simulink model "PlaneFlexSim"  (Simulink 7.4)
settings: Solver=ode23tb  StartTime=0  StopTime=10  FixedStep=ts  MaxStep=.01  RelTol=1e-3
model workspace (MAT data in the model file):
  ts : num (value not decoded)
values from neighbouring files (symbols this model uses):
  simRunner = SimRunner('simRunner')    [testSimRunner.m]
libraries: mblibv1 x23, FlutterLib x8, simulink x1
settings Model: Creator=cstephen  ModifiedByFormat=Rafal  LastModifiedBy=Rafal  ExtModeArmWhenConnect=off  BufferReuse=off
settings DataIOCC: LimitDataPoints=off  SaveOutput=off  SaveTime=off  SignalLoggingName=sigsOut
settings OptimizationCC: BlockReduction=off  InlineParams=on  OptimizeBlockIOStorage=off  BufferReuse=off  EnforceIntegerDowncast=off  ExpressionFolding=off  FoldNonRolledExpr=off  LocalBlockOutputs=off  InitFltsAndDblsToZero=on
settings DebuggingCC: AlgebraicLoopMsg=none  SaveWithParameterizedLinksMsg=none  SignalResolutionControl=TryResolveAllWithWarning  SolverPrmCheckMsg=none  MultiTaskDSMMsg=warning  MultiTaskCondExecSysMsg=none  UnconnectedInputMsg=none  UnconnectedOutputMsg=none  UnconnectedLineMsg=none  StrictBusMsg=None
settings HardwareCC: TargetUnknown=on
settings RTWCC: SystemTargetFile=xpctarget.tlc  TemplateMakefile=xpc_default_tmf  ProcessScript=xpctarget_make_rtw_hook  IncludeERTFirstTime=on
settings xpcTargetCC: TargetFcnLib=ansi_tfl_tmw.mat  TargetFunctionLibrary=ANSI_C  ParMdlRefBuildCompliant=off  CompOptLevelCompliant=off  PortableWordSizes=off
settings CustomProperty: DataType=string  Value=Real-Time
settings SimMechanicsCC: VisDuringSimulation=on  VisSampleTime=0.1  LastVizWinPosition=[360 278 560 420]  CamPosition=[0;-0.208325;16.8123;]  CamTarget=[0;-0.208325;0.424625;]  CamUpVector=[0;1;0;]  CamHeight=4.41673  VisBackgroundColor=[0.9;0.9;0.95;]  DefaultBodyColor=[1;0;0;]

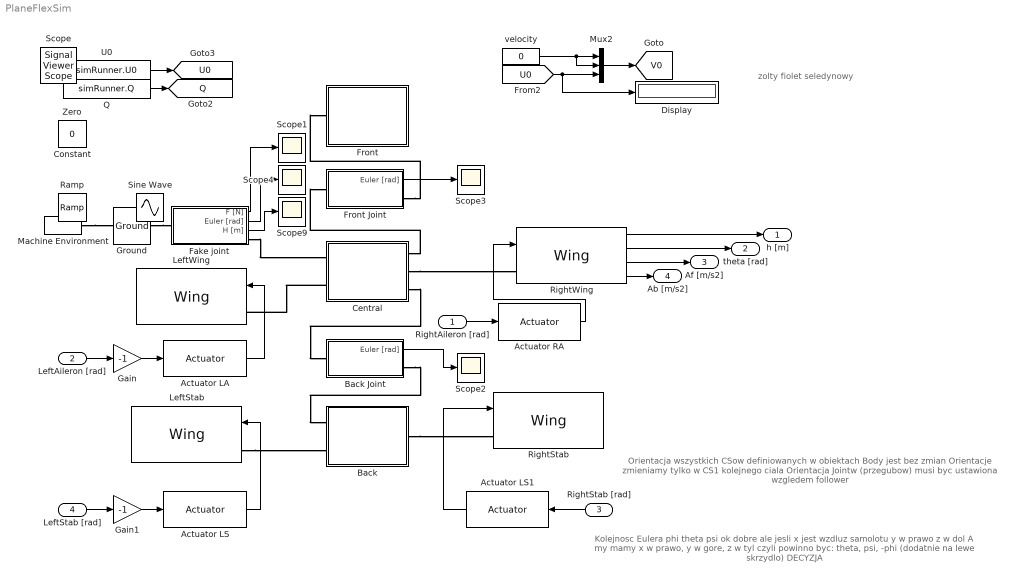
== system PlaneFlexSim ==
  note: Orientacja wszystkich CSow definiowanych
      | w obiektach Body jest bez zmian
      | Orientacje zmieniamy tylko w CS1 kolejnego ciala
      | Orientacja Jointw (przegubow) musi byc ustawiona
      | wzgledem follower
  note: zolty
      | fiolet
      | seledynowy
  note: Kolejnosc Eulera
      | phi theta psi
      | ok dobre ale jesli x jest wzdluz samolotu
      | y w prawo z w dol
      | A my mamy x w prawo, y w gore, z w tyl
      | czyli powinno byc:
      | theta, psi, -phi (dodatnie na lewe skrzydlo)
      | DECYZJA
  RightAileron [rad] : Inport  OutDataType=fixdt(1, 16)  OutScaling=2^0
  LeftAileron [rad] : Inport  Port=2  OutDataType=fixdt(1, 16)  OutScaling=2^0
  RightStab [rad] : Inport  Port=3  OutDataType=fixdt(1, 16)  OutScaling=2^0
  LeftStab [rad] : Inport  Port=4  OutDataType=fixdt(1, 16)  OutScaling=2^0
  Actuator LA : FlutterLib/Actuator  SystemSampleTime=-1  actuator=simRunner.actuator
  Actuator LS : FlutterLib/Actuator  SystemSampleTime=-1  actuator=simRunner.actuator
  Actuator LS1 : FlutterLib/Actuator  SystemSampleTime=-1  actuator=simRunner.actuator
  Actuator RA : FlutterLib/Actuator  SystemSampleTime=-1  actuator=simRunner.actuator
  Back : Subsystem
  Back Joint : Subsystem
  Central : Subsystem
  Display : Display
  Fake joint : Subsystem
  Front : Subsystem
  Front Joint : Subsystem
  Gain : Gain  Gain=-1  ParameterDataType=fixdt(1, 16)  ParameterScaling=2^0  OutDataType=fixdt(1, 16)  OutScaling=2^0
  Gain1 : Gain  Gain=-1  ParameterDataType=fixdt(1, 16)  ParameterScaling=2^0  OutDataType=fixdt(1, 16)  OutScaling=2^0
  Ground : mblibv1/Bodies/Ground  DialogController=MECH.DynMechDlgSource  SystemSampleTime=-1  UpdateFromCAD=off  LeftPortType=env  RightPortType=workingframe  PhysicalDomain=Mechanical  DialogClass=GroundBlock  CoordPosition=[0 0 0]  CoordPositionUnits=m  StateVectorMgrId=-1  MachineId=[0 0]  ShowEnvPort=on
  LeftStab : FlutterLib/Wing  SystemSampleTime=-1  wing=simRunner.stabParams  wingOrientation=[0 0 210]
  LeftWing : FlutterLib/Wing  SystemSampleTime=-1  wing=simRunner.wingParams  wingOrientation=[0 0 -180]
  Machine Environment : mblibv1/Bodies/Machine Environment  DialogController=MECH.DialogSource  SystemSampleTime=-1  PortType=env  PhysicalDomain=Mechanical  DialogTemplateClass=MECH.MachineEnvironment  SyncWhenCopied=off  Gravity=[0 -simRunner.g 0]  GravityUnits=m/s^2  GravityAsSignal=off  Dimensionality=3D Only  AnalysisType=Forward dynamics  LinearAssemblyTolerance=1e-3  LinearAssemblyToleranceUnits=m  AngularAssemblyTolerance=1e-3  AngularAssemblyToleranceUnits=rad  ConstraintSolverType=Stabilizing  ConstraintRelTolerance=1e-4  ConstraintAbsTolerance=1e-4  UseRobustSingularityHandling=off  RedundancyAnalysisToleranceType=Automatically select tolerance  RedundancyAnalysisTolerance=1e-14  StatePerturbationType=Adaptive  PerturbationSize=1e-3  VisualizeMachine=on  BodyVisualizationType=Use model default body geometries  BodyColorSelMode=Use model default  DefaultBodyColor=[1 0 0]
  Mux2 : Mux  Inputs=3
  Q : Constant  Value=simRunner.Q  OutDataType=sfix(16)  OutScaling=2^0
  RightStab : FlutterLib/Wing  SystemSampleTime=-1  wing=simRunner.stabParams  wingOrientation=[0 0 -30]
  RightWing : FlutterLib/Wing  SystemSampleTime=-1  wing=simRunner.wingParams  wingOrientation=[0 0 0]
  Scope{1..4,9} (5 alike) : Scope
      Scope3 settings: SaveName=ScopeData2
      Scope4 settings: SaveName=ScopeData3
      Scope9 settings: SaveName=ScopeData8
  U0 : Constant  Value=simRunner.U0  OutDataType=sfix(16)  OutScaling=2^0
  velocity : Constant  Value=0  OutDataType=sfix(16)  OutScaling=2^0
  h [m] : Outport  OutDataType=fixdt(1, 16)  OutScaling=2^0
  theta [rad] : Outport  Port=2  OutDataType=fixdt(1, 16)  OutScaling=2^0
  Af [m/s2] : Outport  Port=3  OutDataType=fixdt(1, 16)  OutScaling=2^0
  Ab [m/s2] : Outport  Port=4  OutDataType=fixdt(1, 16)  OutScaling=2^0
  Constant : Constant  IOType=siggen  Value=-1  OutDataType=sfix(16)  OutScaling=2^0
  Ramp : simulink/Sources/Ramp  IOType=siggen  SystemSampleTime=-1  slope=1  start=0  X0=0
  Scope : SignalViewerScope  IOType=viewer  ZoomMode=xonly  LegendLocations="674.3333      275.3333            95            41"  RefreshTime=0.035000
      settings: ShowLegends=on  YMin=-0.0018  YMax=0.0002
  Sine Wave : Sin  IOType=siggen  Amplitude=10  Bias=0  Frequency=5  Phase=pi/2  Samples=10  SampleTime=0  Offset=0
  Zero : Constant  IOType=siggen  Value=0  OutDataType=sfix(16)  OutScaling=2^0
  tag scope: Q=global, U0=global, V0=global
  wires:
  [U0] -> Mux2/3, Display/1
  Mux2/1 -> [V0]
  velocity/1 -> Mux2/1, Mux2/2
  Fake joint/1(F [N]) -> Scope1/1
  Front Joint/1(Euler [rad]) -> Scope3/1
  Back Joint/1(Euler [rad]) -> Scope2/1
  Fake joint/2(Euler [rad]) -> Scope4/1
  RightAileron [rad]/1 -> Actuator RA/1
  LeftStab [rad]/1 -> Gain1/1
  RightStab [rad]/1 -> Actuator LS1/1
  Fake joint/3(H [m]) -> Scope9/1
  U0/1 -> [U0]
  Q/1 -> [Q]
  Actuator RA/1 -> RightWing/1
  RightWing/2 -> theta [rad]/1
  RightWing/1 -> h [m]/1
  RightWing/3 -> Af [m/s2]/1
  RightWing/4 -> Ab [m/s2]/1
  LeftAileron [rad]/1 -> Gain/1
  Actuator LA/1 -> LeftWing/1
  Actuator LS/1 -> LeftStab/1
  Actuator LS1/1 -> RightStab/1
  Gain/1 -> Actuator LA/1
  Gain1/1 -> Actuator LS/1
  connections:
  Machine Environment/RConn1 -- Ground/LConn1
  Ground/RConn1 -- Fake joint/LConn1
  Fake joint/RConn1 -- Central/LConn1
  Central/RConn3 -- Back Joint/LConn1
  Back Joint/RConn1 -- Back/LConn1
  Central/RConn1 -- Front Joint/LConn1
  Front Joint/RConn1 -- Front/LConn1
  Back/RConn1 -- RightStab/LConn1
  LeftStab/LConn1 -- Back/LConn2
  Central/LConn2 -- LeftWing/LConn1
  Central/RConn2 -- RightWing/LConn1

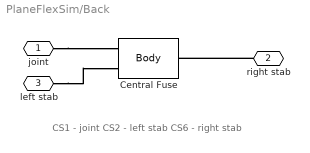
== system PlaneFlexSim/Back ==
  note: CS1 - joint
      | CS2 - left stab
      | CS6 - right stab
  Central Fuse : mblibv1/Bodies/Body  DialogController=MECH.DynMechDlgSource  PhysicalDomain=mechanical  SubClassName=Unknown  LeftPortType=workingframe  RightPortType=workingframe  LConnTagsString=CS1|CS2  RConnTagsString=CS6  UpdateFromCAD=off  DialogClass=MechanicalBodyBlock  Mass=simRunner.fuse.Back.Mass  MassUnits=kg  InertiaUnits=kg*m^2  Inertia=simRunner.fuse.Back.Inertia  Shape=Cylinder  ShapeDims=[1 1]  ShapeUnits=m  ShapeUse=false  Density=1  DensityUnits=kg/m^3  DensityUse=false  GraphicsMode=MACHINE_DEFAULT  BodyColorSelMode=MACHINE_DEFAULT  BodyColor=[1 0 0]  AttachedToCS=CG  CG=Left$CG$simRunner.fuse.Back.CG$CS1$CS1$m$[0 0 0]$Euler X-Y-Z$deg$CS1$false$none  WorkingFrames=Left$CS1$[0 0 0]$Adjoining$Adjoining$m$[0 0 0]$Euler X-Y-Z$deg$Adjoining$true$none#Right$CS6$[0 0 3.1]$CS1$CS1$m$[0 0 0]$Euler X-Y-Z$deg$CS1$true$none#Left$CS2$[0 0 3.1]$CS1$CS1$m$[0 0 0]$Euler X-Y-Z$deg$CS1$true$none#Left$CS5$[-0.4 0 0]$CS1$CS1$m$[0 0 0]$Euler X-Y-Z$deg$CS1$false$none#Left$CS3$[0 0.8 0]$CS1$CS1$m$[0 0 0]$Euler X-Y-Z$deg$CS1$false$none#Left$CS9$[0.4 0 0]$CS1$CS1$m$[0 0 0]$Euler X-Y-Z$deg$CS1$false$none#Left$CS8$[0 -0.2 0]$CS1$CS1$m$[0 0 0]$Euler X-Y-Z$deg$CS1$false$none#Left$CS10$[-0.2 0 3.6]$CS1$CS1$m$[0 0 0]$Euler X-Y-Z$deg$CS1$false$none#Left$CS13$[0 0.2 3.6]$CS1$CS1$m$[0 0 0]$Euler X-Y-Z$deg$CS1$false$none#Left$CS12$[0.2 0 3.6]$CS1$CS1$m$[0 0 0]$Euler X-Y-Z$deg$CS1$false$none#Left$CS11$[0 -0.1 3.6]$CS1$CS1$m$[0 0 0]$Euler X-Y-Z$deg$CS1$false$none  CGPos=simRunner.fuse.Back.CG  CGRot=[0 0 0]  CS0Pos=[]  CS0Rot=[]  CS1Pos=[0 0 0]  CS1Rot=[0 0 0]  CS2Pos=[0 0 3.1]  CS2Rot=[0 0 0]  CS3Pos=[0 0.8 0]  CS3Rot=[0 0 0]  CS4Pos=[]  CS4Rot=[]  CS5Pos=[-0.4 0 0]  CS5Rot=[0 0 0]  CS6Pos=[0 0 3.1]  CS6Rot=[0 0 0]  CS7Pos=[]  CS7Rot=[]  CS8Pos=[0 -0.2 0]  CS8Rot=[0 0 0]  CS9Pos=[0.4 0 0]  CS9Rot=[0 0 0]  CS10Pos=[-0.2 0 3.6]  CS10Rot=[0 0 0]  CS11Pos=[0 -0.1 3.6]  CS11Rot=[0 0 0]  CS12Pos=[0.2 0 3.6]  CS12Rot=[0 0 0]  CS13Pos=[0 0.2 3.6]  CS13Rot=[0 0 0]  CS14Pos=[]  CS14Rot=[]  CS15Pos=[]  CS15Rot=[]  CS16Pos=[]  CS16Rot=[]  CS17Pos=[]  CS17Rot=[]  CS18Pos=[]  CS18Rot=[]  CS19Pos=[]  CS19Rot=[]  CS20Pos=[]  CS20Rot=[]
  joint : PMIOPort  Port=1  Side=Left
  right stab : PMIOPort  Port=2  Side=Right
  left stab : PMIOPort  Port=3  Side=Left
  connections:
  right stab/RConn1 -- Central Fuse/RConn1
  joint/RConn1 -- Central Fuse/LConn1
  left stab/RConn1 -- Central Fuse/LConn2

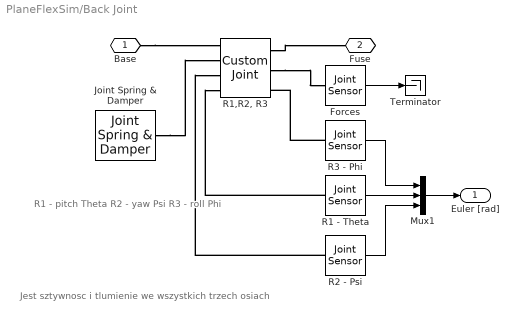
== system PlaneFlexSim/Back Joint ==
  note: R1 - pitch Theta
      | R2 - yaw Psi
      | R3 - roll Phi
  note: Jest sztywnosc i
      | tlumienie
      | we wszystkich trzech
      | osiach
  Forces : mblibv1/Sensors &  Actuators/Joint Sensor  DialogController=MECH.DynMechDlgSource  SystemSampleTime=-1  UpdateFromCAD=off  PhysicalDomain=Mechanical  PortType=blob  Muxed=on  Pose=off  Angle=off  AngleUnits=rad  ArcVelocity=off  ArcVelocityUnits=rad/s  ArcAcceleration=off  ArcAccelerationUnits=deg/s^2  CoordPosition=on  CoordPositionUnits=m  Velocity=off  VelocityUnits=m/s  Acceleration=off  AccelerationUnits=m/s^2  Quaternion=on  QuaternionDT=off  QuaternionDDT=off  QuaternionUnits=off  OutputVector=[1]  ActiveIO=on  Width=3  DialogClass=MechanicalSensorBlock  Primitive=R1  Force=off  ForceUnits=N  Torque=off  TorqueUnits=N*m  ReferenceFrame=Absolute (World)  ReactionSensedSide=Base  ReactionReferenceFrame=Absolute (World)  ReactionForce=on  ReactionForceUnits=N  ReactionMoment=off  ReactionMomentUnits=N*m
  Joint Spring & Damper : mblibv1/Force  Elements/Joint Spring & Damper  DialogController=MECH.DynMechDlgSource  SystemSampleTime=-1  UpdateFromCAD=off  DialogClass=JointSpringDamper  JFEParameters=P1$false$0$0$0$m$m/s$N$deg$deg/s$N*m#P2$false$0$0$0$m$m/s$N$deg$deg/s$N*m#P3$false$0$0$0$m$m/s$N$deg$deg/s$N*m#R1$true$simRunner.fuse.K.K_theta$simRunner.fuse.K.Zeta_theta$0$m$m/s$N$deg$deg/s$N*m#R2$true$simRunner.fuse.K.K_psi$simRunner.fuse.K.Zeta_psi$0$m$m/s$N$deg$deg/s$N*m#R3$true$simRunner.fuse.K.K_phi$simRunner.fuse.K.Zeta_phi$0$m$m/s$N$deg$deg/s$N*m#S$false$0$0$0$m$m/s$N$deg$deg/s$N*m
  Mux1 : Mux  Inputs=3
  R1 - Theta : mblibv1/Sensors &  Actuators/Joint Sensor  DialogController=MECH.DynMechDlgSource  SystemSampleTime=-1  UpdateFromCAD=off  PhysicalDomain=Mechanical  PortType=blob  Muxed=on  Pose=off  Angle=on  AngleUnits=rad  ArcVelocity=off  ArcVelocityUnits=rad/s  ArcAcceleration=off  ArcAccelerationUnits=deg/s^2  CoordPosition=on  CoordPositionUnits=m  Velocity=off  VelocityUnits=m/s  Acceleration=off  AccelerationUnits=m/s^2  Quaternion=on  QuaternionDT=off  QuaternionDDT=off  QuaternionUnits=off  OutputVector=[1]  ActiveIO=on  Width=1  DialogClass=MechanicalSensorBlock  Primitive=R1  Force=off  ForceUnits=N  Torque=off  TorqueUnits=N*m  ReferenceFrame=Absolute (World)  ReactionSensedSide=Base  ReactionReferenceFrame=Absolute (World)  ReactionForce=off  ReactionForceUnits=N  ReactionMoment=off  ReactionMomentUnits=N*m
  "R1,R2, R3" : mblibv1/Joints/Custom Joint  DialogController=MECH.DynMechDlgSource  PhysicalDomain=mechanical  SubClassName=custom_joint  LeftPortType=blob  RightPortType=blob  LConnTagsString=__newl0|SA1|SA2|SA3  RConnTagsString=__newr0|SA1|SA2  UpdateFromCAD=off  NumSAPorts=5  CutJoint=off  MarkAsCut=off  Primitives=prismatic  PrimitiveProps=R1$Follower$[1 0 0]$revolute#R2$Follower$[0 1 0]$Revolute#R3$Follower$[0 0 1]$Revolute  DialogClass=JointBlock  R1Axis=[1 0 0]  R2Axis=[0 1 0]  R3Axis=[0 0 1]  P1Axis=[]  P2Axis=[]  P3Axis=[]  SAxis=[]
  R2 - Psi : mblibv1/Sensors &  Actuators/Joint Sensor  DialogController=MECH.DynMechDlgSource  SystemSampleTime=-1  UpdateFromCAD=off  PhysicalDomain=Mechanical  PortType=blob  Muxed=on  Pose=off  Angle=on  AngleUnits=rad  ArcVelocity=off  ArcVelocityUnits=rad/s  ArcAcceleration=off  ArcAccelerationUnits=deg/s^2  CoordPosition=on  CoordPositionUnits=m  Velocity=off  VelocityUnits=m/s  Acceleration=off  AccelerationUnits=m/s^2  Quaternion=on  QuaternionDT=off  QuaternionDDT=off  QuaternionUnits=off  OutputVector=[1]  ActiveIO=on  Width=1  DialogClass=MechanicalSensorBlock  Primitive=R2  Force=off  ForceUnits=N  Torque=off  TorqueUnits=N*m  ReferenceFrame=Absolute (World)  ReactionSensedSide=Base  ReactionReferenceFrame=Absolute (World)  ReactionForce=off  ReactionForceUnits=N  ReactionMoment=off  ReactionMomentUnits=N*m
  R3 - Phi : mblibv1/Sensors &  Actuators/Joint Sensor  DialogController=MECH.DynMechDlgSource  SystemSampleTime=-1  UpdateFromCAD=off  PhysicalDomain=Mechanical  PortType=blob  Muxed=on  Pose=off  Angle=on  AngleUnits=rad  ArcVelocity=off  ArcVelocityUnits=rad/s  ArcAcceleration=off  ArcAccelerationUnits=deg/s^2  CoordPosition=on  CoordPositionUnits=m  Velocity=off  VelocityUnits=m/s  Acceleration=off  AccelerationUnits=m/s^2  Quaternion=on  QuaternionDT=off  QuaternionDDT=off  QuaternionUnits=off  OutputVector=[1]  ActiveIO=on  Width=1  DialogClass=MechanicalSensorBlock  Primitive=R3  Force=off  ForceUnits=N  Torque=off  TorqueUnits=N*m  ReferenceFrame=Absolute (World)  ReactionSensedSide=Base  ReactionReferenceFrame=Absolute (World)  ReactionForce=off  ReactionForceUnits=N  ReactionMoment=off  ReactionMomentUnits=N*m
  Terminator : Terminator
  Base : PMIOPort  Port=1  Side=Left
  Fuse : PMIOPort  Port=2  Side=Right
  Euler [rad] : Outport  OutDataType=fixdt(1, 16)  OutScaling=2^0
  wires:
  Mux1/1 -> Euler [rad]/1
  R2 - Psi/1 -> Mux1/3
  R1 - Theta/1 -> Mux1/2
  R3 - Phi/1 -> Mux1/1
  Forces/1 -> Terminator/1
  connections:
  R1 - Theta/LConn1 -- "R1,R2, R3"/LConn4
  R3 - Phi/LConn1 -- "R1,R2, R3"/RConn3
  Base/RConn1 -- "R1,R2, R3"/LConn1
  "R1,R2, R3"/RConn1 -- Fuse/RConn1
  "R1,R2, R3"/RConn2 -- Forces/LConn1
  R2 - Psi/LConn1 -- "R1,R2, R3"/LConn3
  Joint Spring & Damper/LConn1 -- "R1,R2, R3"/LConn2

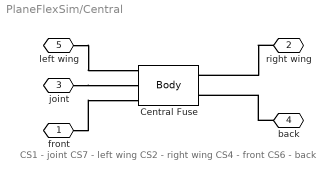
== system PlaneFlexSim/Central ==
  note: CS1 - joint
      | CS7 - left wing
      | CS2 - right wing
      | CS4 - front
      | CS6 - back
  Central Fuse : mblibv1/Bodies/Body  DialogController=MECH.DynMechDlgSource  PhysicalDomain=mechanical  SubClassName=Unknown  LeftPortType=workingframe  RightPortType=workingframe  LConnTagsString=CS7|CS1|CS4  RConnTagsString=CS2|CS6  UpdateFromCAD=off  DialogClass=MechanicalBodyBlock  Mass=simRunner.fuse.Central.Mass  MassUnits=kg  InertiaUnits=kg*m^2  Inertia=simRunner.fuse.Central.Inertia  Shape=Cylinder  ShapeDims=[1 1]  ShapeUnits=m  ShapeUse=false  Density=1  DensityUnits=kg/m^3  DensityUse=false  GraphicsMode=MACHINE_DEFAULT  BodyColorSelMode=MACHINE_DEFAULT  BodyColor=[1 0 0]  AttachedToCS=CG  CG=Left$CG$[0 0 0.3]$CS1$CS1$m$[0 0 0]$Euler X-Y-Z$deg$CS1$false$none  WorkingFrames=Left$CS7$[-0.4 0 0]$CS1$CS1$m$[0 0 0]$Euler X-Y-Z$deg$CS1$true$none#Left$CS1$[0 0 0]$Adjoining$Adjoining$m$[5 0 0]$Euler X-Y-Z$deg$Adjoining$true$none#Right$CS2$[0.4 0 0]$CS1$CS1$m$[0 0 0]$Euler X-Y-Z$deg$CS1$true$none#Left$CS4$[0 0 -0.3]$CS1$CS1$m$[0 0 0]$Euler X-Y-Z$deg$CS1$true$none#Right$CS6$[0 0 0.9]$CS1$CS1$m$[0 0 0]$Euler X-Y-Z$deg$CS1$true$none#Left$CS5$[-0.4 0 -0.3]$CS1$CS1$m$[0 0 0]$Euler X-Y-Z$deg$CS1$false$none#Left$CS3$[0 0.8 -0.3]$CS1$CS1$m$[0 0 0]$Euler X-Y-Z$deg$CS1$false$none#Left$CS9$[0.4 0 -0.3]$CS1$CS1$m$[0 0 0]$Euler X-Y-Z$deg$CS1$false$none#Left$CS8$[0 -0.2 -0.3]$CS1$CS1$m$[0 0 0]$Euler X-Y-Z$deg$CS1$false$none#Left$CS10$[-0.4 0 0.9]$CS1$CS1$m$[0 0 0]$Euler X-Y-Z$deg$CS1$false$none#Left$CS13$[0 0.8 0.9]$CS1$CS1$m$[0 0 0]$Euler X-Y-Z$deg$CS1$false$none#Left$CS12$[0.4 0 0.9]$CS1$CS1$m$[0 0 0]$Euler X-Y-Z$deg$CS1$false$none#Left$CS11$[0 -0.2 0.9]$CS1$CS1$m$[0 0 0]$Euler X-Y-Z$deg$CS1$false$none  CGPos=[0 0 0.3]  CGRot=[0 0 0]  CS0Pos=[]  CS0Rot=[]  CS1Pos=[0 0 0]  CS1Rot=[5 0 0]  CS2Pos=[0.4 0 0]  CS2Rot=[0 0 0]  CS3Pos=[0 0.8 -0.3]  CS3Rot=[0 0 0]  CS4Pos=[0 0 -0.3]  CS4Rot=[0 0 0]  CS5Pos=[-0.4 0 -0.3]  CS5Rot=[0 0 0]  CS6Pos=[0 0 0.9]  CS6Rot=[0 0 0]  CS7Pos=[-0.4 0 0]  CS7Rot=[0 0 0]  CS8Pos=[0 -0.2 -0.3]  CS8Rot=[0 0 0]  CS9Pos=[0.4 0 -0.3]  CS9Rot=[0 0 0]  CS10Pos=[-0.4 0 0.9]  CS10Rot=[0 0 0]  CS11Pos=[0 -0.2 0.9]  CS11Rot=[0 0 0]  CS12Pos=[0.4 0 0.9]  CS12Rot=[0 0 0]  CS13Pos=[0 0.8 0.9]  CS13Rot=[0 0 0]  CS14Pos=[]  CS14Rot=[]  CS15Pos=[]  CS15Rot=[]  CS16Pos=[]  CS16Rot=[]  CS17Pos=[]  CS17Rot=[]  CS18Pos=[]  CS18Rot=[]  CS19Pos=[]  CS19Rot=[]  CS20Pos=[]  CS20Rot=[]
  front : PMIOPort  Port=1  Side=Right
  right wing : PMIOPort  Port=2  Side=Right
  joint : PMIOPort  Port=3  Side=Left
  back : PMIOPort  Port=4  Side=Right
  left wing : PMIOPort  Port=5  Side=Left
  connections:
  left wing/RConn1 -- Central Fuse/LConn1
  right wing/RConn1 -- Central Fuse/RConn1
  joint/RConn1 -- Central Fuse/LConn2
  back/RConn1 -- Central Fuse/RConn2
  front/RConn1 -- Central Fuse/LConn3

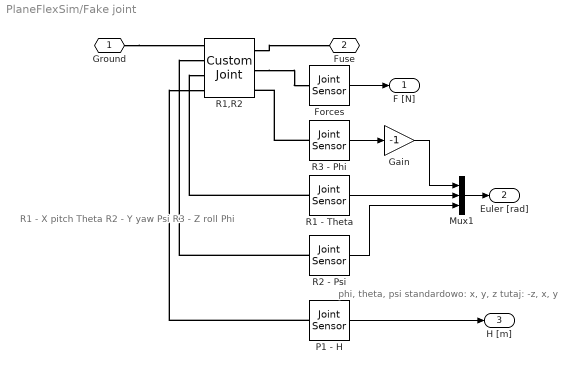
== system PlaneFlexSim/Fake joint ==
  note: R1 - X pitch Theta
      | R2 - Y yaw Psi
      | R3 - Z roll Phi
  note: phi, theta, psi
      | standardowo: x, y, z
      | tutaj: -z, x, y
  Forces : mblibv1/Sensors &  Actuators/Joint Sensor  DialogController=MECH.DynMechDlgSource  SystemSampleTime=-1  UpdateFromCAD=off  PhysicalDomain=Mechanical  PortType=blob  Muxed=on  Pose=off  Angle=off  AngleUnits=rad  ArcVelocity=off  ArcVelocityUnits=rad/s  ArcAcceleration=off  ArcAccelerationUnits=deg/s^2  CoordPosition=on  CoordPositionUnits=m  Velocity=off  VelocityUnits=m/s  Acceleration=off  AccelerationUnits=m/s^2  Quaternion=on  QuaternionDT=off  QuaternionDDT=off  QuaternionUnits=off  OutputVector=[1]  ActiveIO=on  Width=3  DialogClass=MechanicalSensorBlock  Primitive=R1  Force=off  ForceUnits=N  Torque=off  TorqueUnits=N*m  ReferenceFrame=Absolute (World)  ReactionSensedSide=Base  ReactionReferenceFrame=Absolute (World)  ReactionForce=on  ReactionForceUnits=N  ReactionMoment=off  ReactionMomentUnits=N*m
  Gain : Gain  Gain=-1  ParameterDataType=fixdt(1, 16)  ParameterScaling=2^0  OutDataType=fixdt(1, 16)  OutScaling=2^0
  Mux1 : Mux  Inputs=3
  P1 - H : mblibv1/Sensors &  Actuators/Joint Sensor  DialogController=MECH.DynMechDlgSource  SystemSampleTime=-1  UpdateFromCAD=off  PhysicalDomain=Mechanical  PortType=blob  Muxed=on  Pose=off  Angle=off  AngleUnits=rad  ArcVelocity=off  ArcVelocityUnits=rad/s  ArcAcceleration=off  ArcAccelerationUnits=deg/s^2  CoordPosition=on  CoordPositionUnits=m  Velocity=off  VelocityUnits=m/s  Acceleration=off  AccelerationUnits=m/s^2  Quaternion=on  QuaternionDT=off  QuaternionDDT=off  QuaternionUnits=off  OutputVector=[1]  ActiveIO=on  Width=1  DialogClass=MechanicalSensorBlock  Primitive=P1  Force=off  ForceUnits=N  Torque=off  TorqueUnits=N*m  ReferenceFrame=Absolute (World)  ReactionSensedSide=Base  ReactionReferenceFrame=Absolute (World)  ReactionForce=off  ReactionForceUnits=N  ReactionMoment=off  ReactionMomentUnits=N*m
  R1 - Theta : mblibv1/Sensors &  Actuators/Joint Sensor  DialogController=MECH.DynMechDlgSource  SystemSampleTime=-1  UpdateFromCAD=off  PhysicalDomain=Mechanical  PortType=blob  Muxed=on  Pose=off  Angle=on  AngleUnits=rad  ArcVelocity=off  ArcVelocityUnits=rad/s  ArcAcceleration=off  ArcAccelerationUnits=deg/s^2  CoordPosition=on  CoordPositionUnits=m  Velocity=off  VelocityUnits=m/s  Acceleration=off  AccelerationUnits=m/s^2  Quaternion=on  QuaternionDT=off  QuaternionDDT=off  QuaternionUnits=off  OutputVector=[1]  ActiveIO=on  Width=1  DialogClass=MechanicalSensorBlock  Primitive=R1  Force=off  ForceUnits=N  Torque=off  TorqueUnits=N*m  ReferenceFrame=Absolute (World)  ReactionSensedSide=Base  ReactionReferenceFrame=Absolute (World)  ReactionForce=off  ReactionForceUnits=N  ReactionMoment=off  ReactionMomentUnits=N*m
  R1,R2 : mblibv1/Joints/Custom Joint  DialogController=MECH.DynMechDlgSource  PhysicalDomain=mechanical  SubClassName=custom_joint  LeftPortType=blob  RightPortType=blob  LConnTagsString=__newl0|SA1|SA2|SA3  RConnTagsString=__newr0|SA1|SA2  UpdateFromCAD=off  NumSAPorts=5  CutJoint=off  MarkAsCut=off  Primitives=prismatic  PrimitiveProps=R1$Base$[1 0 0]$revolute#R2$Base$[0 1 0]$Revolute#R3$Base$[0 0 1]$Revolute#P1$World$[0 1 0]$Prismatic  DialogClass=JointBlock  R1Axis=[1 0 0]  R2Axis=[0 1 0]  R3Axis=[0 0 1]  P1Axis=[0 1 0]  P2Axis=[]  P3Axis=[]  SAxis=[]
  R2 - Psi : mblibv1/Sensors &  Actuators/Joint Sensor  DialogController=MECH.DynMechDlgSource  SystemSampleTime=-1  UpdateFromCAD=off  PhysicalDomain=Mechanical  PortType=blob  Muxed=on  Pose=off  Angle=on  AngleUnits=rad  ArcVelocity=off  ArcVelocityUnits=rad/s  ArcAcceleration=off  ArcAccelerationUnits=deg/s^2  CoordPosition=on  CoordPositionUnits=m  Velocity=off  VelocityUnits=m/s  Acceleration=off  AccelerationUnits=m/s^2  Quaternion=on  QuaternionDT=off  QuaternionDDT=off  QuaternionUnits=off  OutputVector=[1]  ActiveIO=on  Width=1  DialogClass=MechanicalSensorBlock  Primitive=R2  Force=off  ForceUnits=N  Torque=off  TorqueUnits=N*m  ReferenceFrame=Absolute (World)  ReactionSensedSide=Base  ReactionReferenceFrame=Absolute (World)  ReactionForce=off  ReactionForceUnits=N  ReactionMoment=off  ReactionMomentUnits=N*m
  R3 - Phi : mblibv1/Sensors &  Actuators/Joint Sensor  DialogController=MECH.DynMechDlgSource  SystemSampleTime=-1  UpdateFromCAD=off  PhysicalDomain=Mechanical  PortType=blob  Muxed=on  Pose=off  Angle=on  AngleUnits=rad  ArcVelocity=off  ArcVelocityUnits=rad/s  ArcAcceleration=off  ArcAccelerationUnits=deg/s^2  CoordPosition=on  CoordPositionUnits=m  Velocity=off  VelocityUnits=m/s  Acceleration=off  AccelerationUnits=m/s^2  Quaternion=on  QuaternionDT=off  QuaternionDDT=off  QuaternionUnits=off  OutputVector=[1]  ActiveIO=on  Width=1  DialogClass=MechanicalSensorBlock  Primitive=R3  Force=off  ForceUnits=N  Torque=off  TorqueUnits=N*m  ReferenceFrame=Absolute (World)  ReactionSensedSide=Base  ReactionReferenceFrame=Absolute (World)  ReactionForce=off  ReactionForceUnits=N  ReactionMoment=off  ReactionMomentUnits=N*m
  Ground : PMIOPort  Port=1  Side=Left
  Fuse : PMIOPort  Port=2  Side=Right
  F [N] : Outport  OutDataType=fixdt(1, 16)  OutScaling=2^0
  Euler [rad] : Outport  Port=2  OutDataType=fixdt(1, 16)  OutScaling=2^0
  H [m] : Outport  Port=3  OutDataType=fixdt(1, 16)  OutScaling=2^0
  wires:
  Forces/1 -> F [N]/1
  R1 - Theta/1 -> Mux1/2
  R2 - Psi/1 -> Mux1/3
  Mux1/1 -> Euler [rad]/1
  R3 - Phi/1 -> Gain/1
  Gain/1 -> Mux1/1
  P1 - H/1 -> H [m]/1
  connections:
  R1,R2/RConn2 -- Forces/LConn1
  R1,R2/RConn1 -- Fuse/RConn1
  Ground/RConn1 -- R1,R2/LConn1
  R3 - Phi/LConn1 -- R1,R2/RConn3
  R1 - Theta/LConn1 -- R1,R2/LConn3
  R2 - Psi/LConn1 -- R1,R2/LConn2
  P1 - H/LConn1 -- R1,R2/LConn4

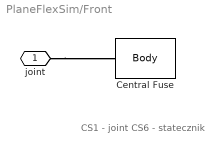
== system PlaneFlexSim/Front ==
  note: CS1 - joint
      | CS6 - statecznik
  Central Fuse : mblibv1/Bodies/Body  DialogController=MECH.DynMechDlgSource  PhysicalDomain=mechanical  SubClassName=Unknown  LeftPortType=workingframe  RightPortType=workingframe  LConnTagsString=CS1  UpdateFromCAD=off  DialogClass=MechanicalBodyBlock  Mass=simRunner.fuse.Front.Mass  MassUnits=kg  InertiaUnits=kg*m^2  Inertia=simRunner.fuse.Front.Inertia  Shape=Cylinder  ShapeDims=[1 1]  ShapeUnits=m  ShapeUse=false  Density=1  DensityUnits=kg/m^3  DensityUse=false  GraphicsMode=MACHINE_DEFAULT  BodyColorSelMode=MACHINE_DEFAULT  BodyColor=[1 0 0]  AttachedToCS=CG  CG=Left$CG$simRunner.fuse.Front.CG$CS1$CS1$m$[0 0 0]$Euler X-Y-Z$deg$CS1$false$none  WorkingFrames=Left$CS1$[0 0 0]$Adjoining$Adjoining$m$[0 0 0]$Euler X-Y-Z$deg$Adjoining$true$none#Left$CS5$[-0.4 0 0]$CS1$CS1$m$[0 0 0]$Euler X-Y-Z$deg$CS1$false$none#Left$CS3$[0 0.8 0]$CS1$CS1$m$[0 0 0]$Euler X-Y-Z$deg$CS1$false$none#Left$CS9$[0.4 0 0]$CS1$CS1$m$[0 0 0]$Euler X-Y-Z$deg$CS1$false$none#Left$CS8$[0 -0.2 0]$CS1$CS1$m$[0 0 0]$Euler X-Y-Z$deg$CS1$false$none#Left$CS10$[-0.5 0 -2.4]$CS1$CS1$m$[0 0 0]$Euler X-Y-Z$deg$CS1$false$none#Left$CS13$[0 0.9 -2.4]$CS1$CS1$m$[0 0 0]$Euler X-Y-Z$deg$CS1$false$none#Left$CS12$[0.5 0 -2.4]$CS1$CS1$m$[0 0 0]$Euler X-Y-Z$deg$CS1$false$none#Left$CS11$[0 -0.2 -2.4]$CS1$CS1$m$[0 0 0]$Euler X-Y-Z$deg$CS1$false$none#Left$CS2$[0 0 -3.4]$CS1$CS1$m$[0 0 0]$Euler X-Y-Z$deg$CS1$false$none  CGPos=simRunner.fuse.Front.CG  CGRot=[0 0 0]  CS0Pos=[]  CS0Rot=[]  CS1Pos=[0 0 0]  CS1Rot=[0 0 0]  CS2Pos=[0 0 -3.4]  CS2Rot=[0 0 0]  CS3Pos=[0 0.8 0]  CS3Rot=[0 0 0]  CS4Pos=[]  CS4Rot=[]  CS5Pos=[-0.4 0 0]  CS5Rot=[0 0 0]  CS6Pos=[]  CS6Rot=[]  CS7Pos=[]  CS7Rot=[]  CS8Pos=[0 -0.2 0]  CS8Rot=[0 0 0]  CS9Pos=[0.4 0 0]  CS9Rot=[0 0 0]  CS10Pos=[-0.5 0 -2.4]  CS10Rot=[0 0 0]  CS11Pos=[0 -0.2 -2.4]  CS11Rot=[0 0 0]  CS12Pos=[0.5 0 -2.4]  CS12Rot=[0 0 0]  CS13Pos=[0 0.9 -2.4]  CS13Rot=[0 0 0]  CS14Pos=[]  CS14Rot=[]  CS15Pos=[]  CS15Rot=[]  CS16Pos=[]  CS16Rot=[]  CS17Pos=[]  CS17Rot=[]  CS18Pos=[]  CS18Rot=[]  CS19Pos=[]  CS19Rot=[]  CS20Pos=[]  CS20Rot=[]
  joint : PMIOPort  Port=1  Side=Left
  connections:
  joint/RConn1 -- Central Fuse/LConn1

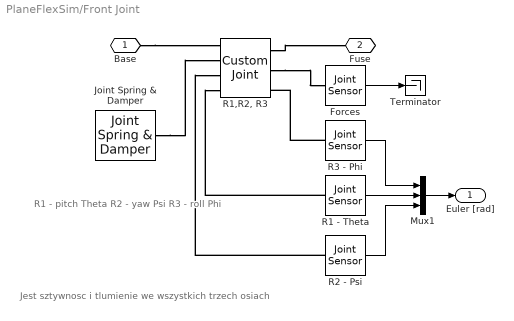
== system PlaneFlexSim/Front Joint ==
  note: Jest sztywnosc i
      | tlumienie
      | we wszystkich trzech
      | osiach
  note: R1 - pitch Theta
      | R2 - yaw Psi
      | R3 - roll Phi
  Forces : mblibv1/Sensors &  Actuators/Joint Sensor  DialogController=MECH.DynMechDlgSource  SystemSampleTime=-1  UpdateFromCAD=off  PhysicalDomain=Mechanical  PortType=blob  Muxed=on  Pose=off  Angle=off  AngleUnits=rad  ArcVelocity=off  ArcVelocityUnits=rad/s  ArcAcceleration=off  ArcAccelerationUnits=deg/s^2  CoordPosition=on  CoordPositionUnits=m  Velocity=off  VelocityUnits=m/s  Acceleration=off  AccelerationUnits=m/s^2  Quaternion=on  QuaternionDT=off  QuaternionDDT=off  QuaternionUnits=off  OutputVector=[1]  ActiveIO=on  Width=3  DialogClass=MechanicalSensorBlock  Primitive=R1  Force=off  ForceUnits=N  Torque=off  TorqueUnits=N*m  ReferenceFrame=Absolute (World)  ReactionSensedSide=Base  ReactionReferenceFrame=Absolute (World)  ReactionForce=on  ReactionForceUnits=N  ReactionMoment=off  ReactionMomentUnits=N*m
  Joint Spring & Damper : mblibv1/Force  Elements/Joint Spring & Damper  DialogController=MECH.DynMechDlgSource  SystemSampleTime=-1  UpdateFromCAD=off  DialogClass=JointSpringDamper  JFEParameters=P1$false$0$0$0$m$m/s$N$deg$deg/s$N*m#P2$false$0$0$0$m$m/s$N$deg$deg/s$N*m#P3$false$0$0$0$m$m/s$N$deg$deg/s$N*m#R1$true$simRunner.fuse.K.K_theta$simRunner.fuse.K.Zeta_theta$0$m$m/s$N$deg$deg/s$N*m#R2$true$simRunner.fuse.K.K_psi$simRunner.fuse.K.Zeta_psi$0$m$m/s$N$deg$deg/s$N*m#R3$true$simRunner.fuse.K.K_phi$simRunner.fuse.K.Zeta_phi$0$m$m/s$N$deg$deg/s$N*m#S$false$0$0$0$m$m/s$N$deg$deg/s$N*m
  Mux1 : Mux  Inputs=3
  R1 - Theta : mblibv1/Sensors &  Actuators/Joint Sensor  DialogController=MECH.DynMechDlgSource  SystemSampleTime=-1  UpdateFromCAD=off  PhysicalDomain=Mechanical  PortType=blob  Muxed=on  Pose=off  Angle=on  AngleUnits=rad  ArcVelocity=off  ArcVelocityUnits=rad/s  ArcAcceleration=off  ArcAccelerationUnits=deg/s^2  CoordPosition=on  CoordPositionUnits=m  Velocity=off  VelocityUnits=m/s  Acceleration=off  AccelerationUnits=m/s^2  Quaternion=on  QuaternionDT=off  QuaternionDDT=off  QuaternionUnits=off  OutputVector=[1]  ActiveIO=on  Width=1  DialogClass=MechanicalSensorBlock  Primitive=R1  Force=off  ForceUnits=N  Torque=off  TorqueUnits=N*m  ReferenceFrame=Absolute (World)  ReactionSensedSide=Base  ReactionReferenceFrame=Absolute (World)  ReactionForce=off  ReactionForceUnits=N  ReactionMoment=off  ReactionMomentUnits=N*m
  "R1,R2, R3" : mblibv1/Joints/Custom Joint  DialogController=MECH.DynMechDlgSource  PhysicalDomain=mechanical  SubClassName=custom_joint  LeftPortType=blob  RightPortType=blob  LConnTagsString=__newl0|SA1|SA2|SA3  RConnTagsString=__newr0|SA1|SA2  UpdateFromCAD=off  NumSAPorts=5  CutJoint=off  MarkAsCut=off  Primitives=prismatic  PrimitiveProps=R1$Follower$[1 0 0]$revolute#R2$Follower$[0 1 0]$Revolute#R3$Follower$[0 0 1]$Revolute  DialogClass=JointBlock  R1Axis=[1 0 0]  R2Axis=[0 1 0]  R3Axis=[0 0 1]  P1Axis=[]  P2Axis=[]  P3Axis=[]  SAxis=[]
  R2 - Psi : mblibv1/Sensors &  Actuators/Joint Sensor  DialogController=MECH.DynMechDlgSource  SystemSampleTime=-1  UpdateFromCAD=off  PhysicalDomain=Mechanical  PortType=blob  Muxed=on  Pose=off  Angle=on  AngleUnits=rad  ArcVelocity=off  ArcVelocityUnits=rad/s  ArcAcceleration=off  ArcAccelerationUnits=deg/s^2  CoordPosition=on  CoordPositionUnits=m  Velocity=off  VelocityUnits=m/s  Acceleration=off  AccelerationUnits=m/s^2  Quaternion=on  QuaternionDT=off  QuaternionDDT=off  QuaternionUnits=off  OutputVector=[1]  ActiveIO=on  Width=1  DialogClass=MechanicalSensorBlock  Primitive=R2  Force=off  ForceUnits=N  Torque=off  TorqueUnits=N*m  ReferenceFrame=Absolute (World)  ReactionSensedSide=Base  ReactionReferenceFrame=Absolute (World)  ReactionForce=off  ReactionForceUnits=N  ReactionMoment=off  ReactionMomentUnits=N*m
  R3 - Phi : mblibv1/Sensors &  Actuators/Joint Sensor  DialogController=MECH.DynMechDlgSource  SystemSampleTime=-1  UpdateFromCAD=off  PhysicalDomain=Mechanical  PortType=blob  Muxed=on  Pose=off  Angle=on  AngleUnits=rad  ArcVelocity=off  ArcVelocityUnits=rad/s  ArcAcceleration=off  ArcAccelerationUnits=deg/s^2  CoordPosition=on  CoordPositionUnits=m  Velocity=off  VelocityUnits=m/s  Acceleration=off  AccelerationUnits=m/s^2  Quaternion=on  QuaternionDT=off  QuaternionDDT=off  QuaternionUnits=off  OutputVector=[1]  ActiveIO=on  Width=1  DialogClass=MechanicalSensorBlock  Primitive=R3  Force=off  ForceUnits=N  Torque=off  TorqueUnits=N*m  ReferenceFrame=Absolute (World)  ReactionSensedSide=Base  ReactionReferenceFrame=Absolute (World)  ReactionForce=off  ReactionForceUnits=N  ReactionMoment=off  ReactionMomentUnits=N*m
  Terminator : Terminator
  Base : PMIOPort  Port=1  Side=Left
  Fuse : PMIOPort  Port=2  Side=Right
  Euler [rad] : Outport  OutDataType=fixdt(1, 16)  OutScaling=2^0
  wires:
  Forces/1 -> Terminator/1
  R3 - Phi/1 -> Mux1/1
  R1 - Theta/1 -> Mux1/2
  R2 - Psi/1 -> Mux1/3
  Mux1/1 -> Euler [rad]/1
  connections:
  Joint Spring & Damper/LConn1 -- "R1,R2, R3"/LConn2
  R2 - Psi/LConn1 -- "R1,R2, R3"/LConn3
  "R1,R2, R3"/RConn2 -- Forces/LConn1
  "R1,R2, R3"/RConn1 -- Fuse/RConn1
  Base/RConn1 -- "R1,R2, R3"/LConn1
  R3 - Phi/LConn1 -- "R1,R2, R3"/RConn3
  R1 - Theta/LConn1 -- "R1,R2, R3"/LConn4
